simulink model "generic_IVS"  (R2024a)
settings: Solver=FixedStepDiscrete  StartTime=0.0  StopTime=inf  FixedStep=0.001  RelTol=1e-3  EnableMultiTasking=on
model workspace (MAT data in the model file):
  APPROACH = [-49.2532697283  17.3349288561; -46.8560638421  15.8416334606; -44.4231792578  15.1936580843; -41.9812023919  14.6008735551; -38.6885385845  14.011429265; -35.362557161  13.6848040706; -32.0241539117  13.5706008465; -28.6853351363  13.5838606667; -25.3485360015  13.6460444059; -22.0129625698  13.7095269564; -18.6780310991  13.7591168284; -15.3435011563  13.7913467501; -12.0092330234  13.8076084687; -8.67511534326  13.8114089093; -6.8448506491  12.6583422471; -4.47592539111  11.2827992448; -2.92924455187  9.69969830294; -1.78711593974  7.70591177107; -1.09138599313  5.37718796468; -0.803989099601  2.06842439311; -0.906382362572  -0.865585434223; -1.11270141424  -3.98989029247; -1.27733374307  -7.2306347051; -1.36238880063  -10.5272651383; -1.39346123589  -13.8192198617; -1.38721126794  -17.0599179815; -1.38183107287  -20.1975764072; -1.38752139042  -23.6949492888; -1.35621758439  -26.7735478705; -1.17180910466  -29.6430044256; -0.636199743841  -32.3528870414; 0.459553855509  -34.8408696641; 1.819228747  -36.6414715196; 2.8  -36.6; 3.8  -36.6; 4.8  -36.6; 5.8  -36.6; 6.8  -36.6]
  LANE_LEN = [284; 276; 267]
  LANE_XY = [59.0003214677 62.3317238784 65.6577746803 68.9711287644 72.2614514234 75.5172879138 77.9296982442 80.3117765819 82.6592727002 84.9682672017 87.2351542049 89.4565910317 ... (1704 elements, 284x2x3)]
  N_LANE = 3
  PARK_OCC = [1 1 1 1 1 1 1 1 1 1 1 1 ... (40000 elements, 200x200)]
  WB = 2.9
  branch_lane = 3
  branch_x = -49.2532697283
  branch_y = 17.3349288561
  cruise_lane = 1
  entrance_x = 6
  entrance_y = -36.6
  lane_width = 3.5
  park_goal = [21.4; -44.3; 1.57079632679]
  toll_lane = 1
  toll_post = 20
  toll_pre = 45
  toll_station = 202.6
  toll_x = -176.17
  toll_y = -85.66
  v_cruise = 11
  v_park = 2.78
  waypoints = [-81.8048181182 -79.1416974235 -76.4199514846 -73.3097017696 -70.5703457405 -67.625901331 -64.4903894371 -61.1945301864 -57.8351626085 -54.4642235015 -51.0966947204 -47.7361432477 ... (1754 elements, 877x2)]
libraries: CarMaker4SL x57, simulink x1
(part 1 of 4)
settings Model: Creator=IPG  LastModifiedBy=gmkk6
settings SolverCC: AlgebraicLoopSolver=TrustRegion
settings DataIOCC: LimitDataPoints=on  SaveFormat=Array  SignalLoggingSaveFormat=ModelDataLogs  ReturnWorkspaceOutputs=off  SignalLoggingName=sigsOut
settings OptimizationCC: BooleanDataType=off  ReuseModelBlockBuffer=off  ExpressionDepthLimit=2147483647  InitFltsAndDblsToZero=on  LifeSpan=inf
settings DebuggingCC: SaveWithParameterizedLinksMsg=none  UnderspecifiedInitializationDetection=Classic  MergeDetectMultiDrivingBlocksExec=none  SignalResolutionControl=TryResolveAllWithWarning  MultiTaskDSMMsg=warning  MultiTaskCondExecSysMsg=none  FcnCallInpInsideContextMsg=warning  UnconnectedInputMsg=warning  UnconnectedOutputMsg=warning  UnconnectedLineMsg=warning  StateNameClashWarn=warning  SFUnexpectedBacktrackingDiag=warning  SFNoUnconditionalDefaultTransitionDiag=warning  ArithmeticOperatorsInVariantConditions=warning
settings HardwareCC: ProdBitPerPointer=32  ProdBitPerSizeT=32  ProdBitPerPtrDiffT=32  ProdLargestAtomicFloat=None  ProdIntDivRoundTo=Undefined  ProdEndianess=Unspecified  ProdWordSize=32  ProdHWDeviceType=32-bit Generic  TargetBitPerPointer=64  TargetBitPerSizeT=64  TargetBitPerPtrDiffT=64  TargetLongLongMode=on  TargetIntDivRoundTo=Zero  TargetEndianess=LittleEndian  TargetWordSize=64  TargetHWDeviceType=MATLAB Host  ProdEqTarget=off
settings ModelReferenceCC: EnableRefExpFcnMdlSchedulingChecks=on  PropagateSignalLabelsOutOfModel=off
settings SFSimCC: SimUseLocalCustomCode=off  CustomCodeUndefinedFunction=UseInterfaceOnly
settings RTWCC: RTWUseLocalCustomCode=off  GPUComputeCapability=3.5  DLArmComputeVersion=19.05
settings CodeAppCC: MaxIdLength=63  StateflowObjectComments=on
settings GRTTargetCC: TargetFcnLib=ansi_tfl_tmw.mat  TargetLangStandard=C89/C90 (ANSI)  CombineOutputUpdateFcns=off  GRTInterface=on
settings ConfigComp: CovMetricSettings=dw  CovSaveCumulativeToWorkspaceVar=on  CovSaveSingleToWorkspaceVar=on  CovExternalEMLEnable=off

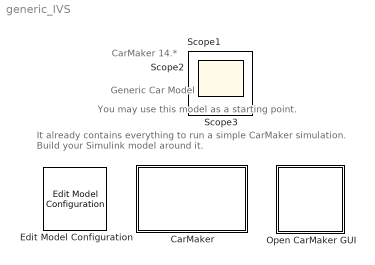
== system generic_IVS ==
  note: Generic Car Model
  note: You may use this model as a starting point.
  note: It already contains everything to run a simple CarMaker simulation.
      | Build your Simulink model around it.
  note: CarMaker 14.*
  CarMaker : Subsystem  TreatAsAtomicUnit=on
      mask Display: image(imread('CarMakerSys.png'));
  Edit Model Configuration : CarMaker4SL/Edit Model Configuration  SFunctionModules=''
  Open CarMaker GUI : Subsystem  LoadFcn=if ~length(which('cmself')), cmenv; end
      settings: OpenFcn=cmblockmagic('gui_fix_display'); CM_Simulink
      mask Display: image(imread('CarMakerGUI.png'));
  Scope1 : Scope
  Scope2 : Scope
  Scope3 : Scope
